simulink model "qamnrzbw"  (Simulink 7.4)
settings: Solver=ode45  StartTime=0.0  StopTime=999999  MaxStep=.05  MinStep=0.0001  RelTol=1e-6  AbsTol=1e-6
undefined symbols (not defined in the file or in its folder): eyediasi, eyesampl, sbiterr
libraries: librnew x3
CloseFcn:
  | closemodcross
settings Model: Creator=gerhard  LastModifiedBy=simulink  ExtModeAutoUpdateStatusClock=off
settings DataIOCC: SaveOutput=off  SaveTime=off  SignalLoggingName=sigsOut
settings OptimizationCC: BlockReduction=off  BooleanDataType=off
settings DebuggingCC: SaveWithParameterizedLinksMsg=none  SignalResolutionControl=TryResolveAllWithWarning  SolverPrmCheckMsg=none  MultiTaskDSMMsg=warning  MultiTaskCondExecSysMsg=none  StrictBusMsg=None
settings HardwareCC: TargetUnknown=on
settings RTWCC: IncludeERTFirstTime=on

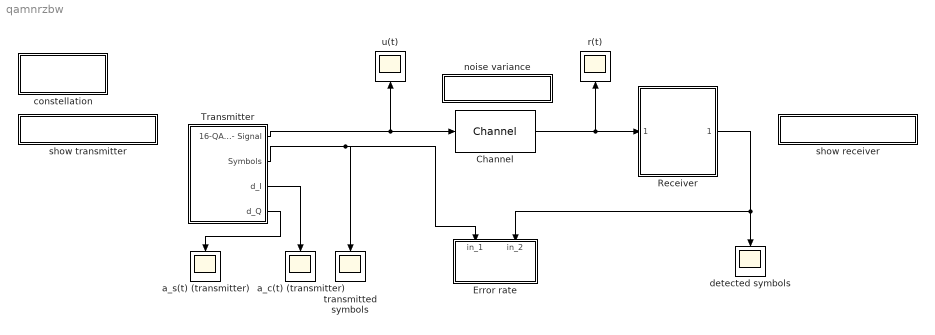
== system qamnrzbw ==
  Channel : librnew/Channel  SystemSampleTime=-1  m=0  variance=0.001  s=12345
  Error rate : Subsystem  LoadFcn=sbiterr([],[],[],'LoadBlock')  StartFcn=sbiterr([],[],[],'Start')  StopFcn=sbiterr([],[],[],'Stop')  mask(Symbol/bit error counter){@1=4, @2=10, @3=1, @4=1}
      mask prompts: @1 "Bit per symbol:"; @2 "Number of digits on display:"; @3 "Delay between 1st port and 2nd port:"; @4 "Sample time (sec):"
      mask help: Use the input data from the 1st port as the reference signal to detect the number of errors and error rate of the 2nd signal.
      mask init:
      | K=@1;num_lin=@2;TDelay=@3;Sample=@4;
      settings: CopyFcn=sbiterr([],[],[],'CopyBlock')  DeleteFcn=sbiterr([],[],[],'DeleteBlock')  NameChangeFcn=sbiterr([],[],[],'NameChange')
      mask Help: The signal from the first port must be a scalar. The second input port can be a vector with a delay to the first port signal. The comparison happens only at the sampling point.
      mask Display: disp('Error\nmeter')
  Receiver : Subsystem
  Transmitter : Subsystem
  a_c(t) (transmitter) : Scope
      settings: TimeRange=25.000000  YMin=-1.5  YMax=1.5  DataFormat=Array
  a_s(t) (transmitter) : Scope
      settings: TimeRange=25.000000  YMin=-1.5  YMax=1.5  DataFormat=Array
  constellation : Subsystem
      settings: OpenFcn=cplotqam(16)
      mask Type: constellation
      mask Display: disp('Signal Space \n Constellation')
  detected symbols : Scope
      settings: TimeRange=25.000000  YMin=-15  YMax=15  DataFormat=Array
  noise variance : Subsystem
      settings: OpenFcn=setnoise
      mask Type: noise
      mask Display: disp('Noise variance')
  r(t) : Scope
      settings: TimeRange=25.000000  YMin=-1.5  YMax=1.5  DataFormat=Array
  show receiver : Subsystem
      settings: OpenFcn=showqamr
      mask Type: open
      mask Display: disp('Receiver')
  show transmitter : Subsystem
      settings: OpenFcn=showqamt
      mask Type: open
      mask Display: disp('Transmitter')
  transmitted symbols : Scope
      settings: TimeRange=25.000000  YMin=-15  YMax=15  DataFormat=Array
  u(t) : Scope
      settings: TimeRange=25.000000  YMin=-1.5  YMax=1.5  DataFormat=Array
  wires:
  Transmitter/1(16-QAM- Signal) -> u(t)/1, Channel/1
  Channel/1 -> Receiver/1(noisy 16-QAM signal), r(t)/1
  Receiver/1(detected symbols) -> detected symbols/1, Error rate/2(in_2)
  Transmitter/4(d_Q) -> a_s(t) (transmitter)/1
  Transmitter/3(d_I) -> a_c(t) (transmitter)/1
  Transmitter/2(Symbols) -> Error rate/1(in_1), transmitted symbols/1

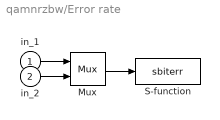
== system qamnrzbw/Error rate ==
  in_1 : Inport  OutDataType=sfix(16)  OutScaling=2^0
  in_2 : Inport  Port=2  OutDataType=sfix(16)  OutScaling=2^0
  Mux : Mux  Inputs=2
  S-function : S-Function  FunctionName=sbiterr  Parameters=num_lin, K, TDelay, Sample  EnableBusSupport=off
  wires:
  Mux/1 -> S-function/1
  in_1/1 -> Mux/1
  in_2/1 -> Mux/2

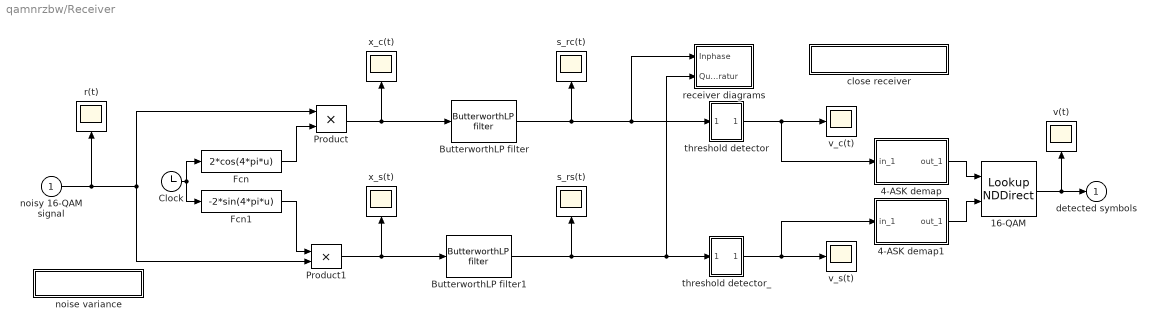
== system qamnrzbw/Receiver ==
  noisy 16-QAM signal : Inport  OutDataType=sfix(16)  OutScaling=2^0
  16-QAM : LookupNDDirect  Table=[0 1 2 3; 4 5 6 7; 8 9 10 11; 12 13 14 15]
  4-ASK demap : Subsystem  mask(MASK demapping){N=4, td=[1, .9]}
      mask prompts: N "M-ary number (digit integers in ranger [0, M-1]):"; td "Output symbol interval and offset (sec):"
      mask help:
      | Reverse the MASK mapping process
      | Convert [-1 1] analog signal to [0, M-1] symbols.
      mask init:
      | Ac=1;sft=[0:N-1]*Ac*2/(N-1)-Ac;
      mask Help: This block demaps a MASK mapped signal back to digit symbols. You can place this block after a amplitude demodulation block. The input of this block is an analog signal in the range [-1, 1]. The demodulation decides the closest integer fitting in [0,M-1] range. When the input symbol interval is a two-elements vector, the second element is offset. The default offset value is 0.
      mask Display: disp('MASK\ndemapping')
  4-ASK demap1 : Subsystem  mask(MASK demapping){N=4, td=[1, .9]}
      mask prompts: N "M-ary number (digit integers in ranger [0, M-1]):"; td "Output symbol interval and offset (sec):"
      mask help:
      | Reverse the MASK mapping process
      | Convert [-1 1] analog signal to [0, M-1] symbols.
      mask init:
      | Ac=1;sft=[0:N-1]*Ac*2/(N-1)-Ac;
      mask Help: This block demaps a MASK mapped signal back to digit symbols. You can place this block after a amplitude demodulation block. The input of this block is an analog signal in the range [-1, 1]. The demodulation decides the closest integer fitting in [0,M-1] range. When the input symbol interval is a two-elements vector, the second element is offset. The default offset value is 0.
      mask Display: disp('MASK\ndemapping')
  ButterworthLP filter : librnew/ButterworthLP filter  SystemSampleTime=-1  n=4  MaskParam1=5
  ButterworthLP filter1 : librnew/ButterworthLP filter  SystemSampleTime=-1  n=4  MaskParam1=5
  Clock : Clock
      settings: Decimation=10
  Fcn : Fcn  Expr=2*cos(4*pi*u)
  Fcn1 : Fcn  Expr=-2*sin(4*pi*u)
  Product : Product  OutDataType=sfix(16)  OutScaling=2^0  SaturateOnIntegerOverflow=on  InputSameDT=on  OutDataTypeStr=Inherit: Same as first input
  Product1 : Product  OutDataType=sfix(16)  OutScaling=2^0  SaturateOnIntegerOverflow=on  InputSameDT=on  OutDataTypeStr=Inherit: Same as first input
  close receiver : Subsystem
      settings: OpenFcn=closqamr
      mask Type: close
      mask Display: disp('close receiver')
  noise variance : Subsystem
      settings: OpenFcn=setnoise
      mask Type: noise
      mask Display: disp('Noise variance')
  r(t) : Scope
      settings: TimeRange=25.000000  YMin=-1.500000  YMax=1.500000  DataFormat=Array
  receiver diagrams : Subsystem  mask(2D-Diagrams){starttime=1, anzahl=40, offset=0.075}
      mask prompts: starttime "Plot start time:"; anzahl "Samples per time slot (2*T):"; offset "Decision offset:"
      mask help: Eye pattern, signal space trajectory and scatter plot
      mask init:
      | [x, y] = srcsicon(10);
      mask Display: plot(0,0,100,100,x,y)
  s_rc(t) : Scope
      settings: TimeRange=25.000000  YMin=-1.500000  YMax=1.500000  DataFormat=Array
  s_rs(t) : Scope
      settings: TimeRange=25.000000  YMin=-1.500000  YMax=1.500000  DataFormat=Array
  threshold detector : Subsystem
  threshold detector_ : Subsystem
  v(t) : Scope
      settings: TimeRange=25.000000  YMin=-15.000000  YMax=15.000000  DataFormat=Array
  v_c(t) : Scope
      settings: TimeRange=25.000000  YMin=-1.500000  YMax=1.500000  DataFormat=Array
  v_s(t) : Scope
      settings: TimeRange=25.000000  YMin=-1.500000  YMax=1.500000  DataFormat=Array
  x_c(t) : Scope
      settings: TimeRange=25.000000  YMin=-1.500000  YMax=1.500000  DataFormat=Array
  x_s(t) : Scope
      settings: TimeRange=25.000000  YMin=-1.500000  YMax=1.500000  DataFormat=Array
  detected symbols : Outport
  wires:
  Clock/1 -> Fcn/1, Fcn1/1
  Product/1 -> x_c(t)/1, ButterworthLP filter/1
  Product1/1 -> x_s(t)/1, ButterworthLP filter1/1
  noisy 16-QAM signal/1 -> r(t)/1, Product/1, Product1/2
  Fcn1/1 -> Product1/1
  Fcn/1 -> Product/2
  ButterworthLP filter/1 -> s_rc(t)/1, receiver diagrams/1(Inphase), threshold detector/1(in_1)
  ButterworthLP filter1/1 -> s_rs(t)/1, receiver diagrams/2(Quadratur), threshold detector_/1(in_1)
  threshold detector/1(out_1) -> v_c(t)/1, 4-ASK demap/1(in_1)
  threshold detector_/1(out_1) -> v_s(t)/1, 4-ASK demap1/1(in_1)
  4-ASK demap/1(out_1) -> 16-QAM/1
  4-ASK demap1/1(out_1) -> 16-QAM/2
  16-QAM/1 -> detected symbols/1, v(t)/1

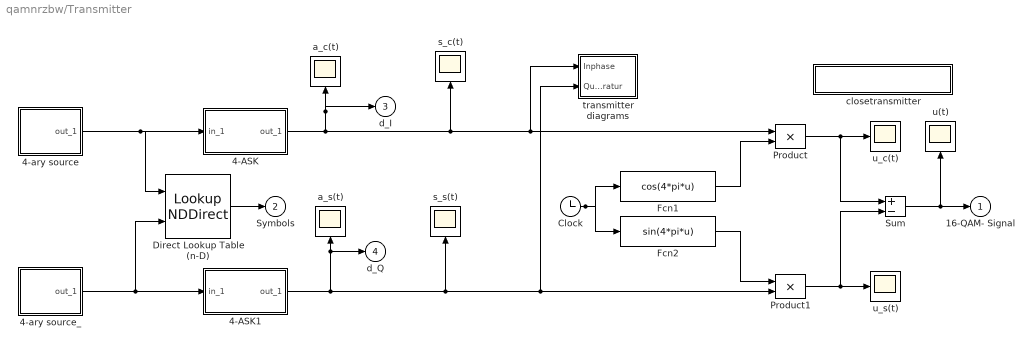
== system qamnrzbw/Transmitter ==
  4-ASK : Subsystem  mask(M-ASK mapping){N=4, td=1}
      mask prompts: N "M-ary number (input integers in range [0, M-1]):"; td "Input symbol interval and offset (sec):"
      mask help:
      | Map a digital symbol onto an analog
      | signal in the range [-1, 1] using M-ary
      | amplitude shift keying modulation mapping.
      mask init:
      | Ac=1;Kc=Ac*2/(N-1);
      mask Help: This block maps an input digit signal onto a signal in the range [-1, 1]. The coded signal can be modulated using analog\nmodulation blocks. Input digits are in the range [0, M-1], where M is the M-ary number. The input symbol interval can be a two-element vector with the second element being offset. The default value offset is 0. Use the MODMAP function to see the constellation.
      mask Display: disp('MASK\nmapping')
  4-ASK1 : Subsystem  mask(M-ASK mapping){N=4, td=1}
      mask prompts: N "M-ary number (input integers in range [0, M-1]):"; td "Input symbol interval and offset (sec):"
      mask help:
      | Map a digital symbol onto an analog
      | signal in the range [-1, 1] using M-ary
      | amplitude shift keying modulation mapping.
      mask init:
      | Ac=1;Kc=Ac*2/(N-1);
      mask Help: This block maps an input digit signal onto a signal in the range [-1, 1]. The coded signal can be modulated using analog\nmodulation blocks. Input digits are in the range [0, M-1], where M is the M-ary number. The input symbol interval can be a two-element vector with the second element being offset. The default value offset is 0. Use the MODMAP function to see the constellation.
      mask Display: disp('MASK\nmapping')
  4-ary source : Subsystem  mask(Read from workspace){@1=randint(2000,1,4), @2=1, @3=1, @4=1}
      mask prompts: @1 "Variable (column_number=block_output_length):"; @2 "Data output sample time (sec):"; @3 "Repeat flag (1: repeat read, 0: output zeros after eof)."; @4 "Initial output:"
      mask help:
      | Read from a workspace variable at
      | sampling time point.
      mask init:
      | var=@1;td=@2;ts=td(1);if (length(td)>=2),off=td(2);else off=0;end;cyc=@3;ini=@4;[x,y]=srcsicon(7);
      mask Help: This block reads from a workspace variable at a given sample time. The column number is the block output vector length. When the simulation reaches the end of the variable (eof), the block will cyclically output from the first row of the variable or output zeros based on the repeat flag entree.
      mask Display: plot(0,0,100,100,x,y);disp('Rd wksp')
  4-ary source_ : Subsystem  mask(Read from workspace){@1=randint(2000,1,4), @2=1, @3=1, @4=1}
      mask prompts: @1 "Variable (column_number=block_output_length):"; @2 "Data output sample time (sec):"; @3 "Repeat flag (1: repeat read, 0: output zeros after eof)."; @4 "Initial output:"
      mask help:
      | Read from a workspace variable at
      | sampling time point.
      mask init:
      | var=@1;td=@2;ts=td(1);if (length(td)>=2),off=td(2);else off=0;end;cyc=@3;ini=@4;[x,y]=srcsicon(7);
      mask Help: This block reads from a workspace variable at a given sample time. The column number is the block output vector length. When the simulation reaches the end of the variable (eof), the block will cyclically output from the first row of the variable or output zeros based on the repeat flag entree.
      mask Display: plot(0,0,100,100,x,y);disp('Rd wksp')
  Clock : Clock
      settings: Decimation=10
  Direct Lookup Table (n-D) : LookupNDDirect  Table=[0 1 2 3; 4 5 6 7; 8 9 10 11; 12 13 14 15]
  Fcn1 : Fcn  Expr=cos(4*pi*u)
  Fcn2 : Fcn  Expr=sin(4*pi*u)
  Product : Product  OutDataType=sfix(16)  OutScaling=2^0  SaturateOnIntegerOverflow=on  InputSameDT=on  OutDataTypeStr=Inherit: Same as first input
  Product1 : Product  OutDataType=sfix(16)  OutScaling=2^0  SaturateOnIntegerOverflow=on  InputSameDT=on  OutDataTypeStr=Inherit: Same as first input
  Sum : Sum  Inputs=+-  OutDataType=sfix(16)  OutScaling=2^0  SaturateOnIntegerOverflow=on  InputSameDT=on  OutDataTypeStr=Inherit: Same as first input
  a_c(t) : Scope
      settings: TimeRange=25.000000  YMin=-1.500000  YMax=1.500000  DataFormat=Array
  a_s(t) : Scope
      settings: TimeRange=25.000000  YMin=-1.500000  YMax=1.500000  DataFormat=Array
  closetransmitter : Subsystem
      settings: OpenFcn=closetra
      mask Type: close
      mask Display: disp('Close transmitter')
  s_c(t) : Scope
      settings: TimeRange=25.000000  YMin=-1.500000  YMax=1.500000  DataFormat=Array
  s_s(t) : Scope
      settings: TimeRange=25.000000  YMin=-1.500000  YMax=1.500000  DataFormat=Array
  transmitter diagrams : Subsystem  mask(2D-Diagrams){starttime=0, anzahl=40, offset=0}
      mask prompts: starttime "Plot start time:"; anzahl "Samples per time slot (2*T):"; offset "Decision offset:"
      mask help: Eye pattern, signal space trajectory and scatter plot
      mask init:
      | [x, y] = srcsicon(10);
      mask Display: plot(0,0,100,100,x,y)
  u(t) : Scope
      settings: TimeRange=25.000000  YMin=-1.500000  YMax=1.500000  DataFormat=Array
  u_c(t) : Scope
      settings: TimeRange=25.000000  YMin=-1.500000  YMax=1.500000  DataFormat=Array
  u_s(t) : Scope
      settings: TimeRange=25.000000  YMin=-1.500000  YMax=1.500000  DataFormat=Array
  16-QAM- Signal : Outport
  Symbols : Outport  Port=2
  d_I : Outport  Port=3
  d_Q : Outport  Port=4
  wires:
  Product1/1 -> u_s(t)/1, Sum/2
  Product/1 -> u_c(t)/1, Sum/1
  Clock/1 -> Fcn2/1, Fcn1/1
  Fcn1/1 -> Product/2
  Fcn2/1 -> Product1/1
  Sum/1 -> u(t)/1, 16-QAM- Signal/1
  4-ary source/1(out_1) -> 4-ASK/1(in_1), Direct Lookup Table (n-D)/1
  Direct Lookup Table (n-D)/1 -> Symbols/1
  4-ASK/1(out_1) -> a_c(t)/1, d_I/1, Product/1, transmitter diagrams/1(Inphase), s_c(t)/1
  4-ASK1/1(out_1) -> a_s(t)/1, d_Q/1, s_s(t)/1, Product1/2, transmitter diagrams/2(Quadratur)
  4-ary source_/1(out_1) -> 4-ASK1/1(in_1), Direct Lookup Table (n-D)/2

== system qamnrzbw/constellation ==

== system qamnrzbw/noise variance ==

== system qamnrzbw/show receiver ==

== system qamnrzbw/show transmitter ==

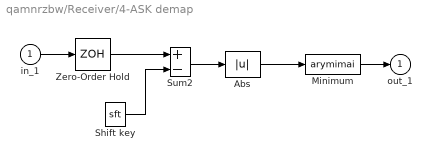
== system qamnrzbw/Receiver/4-ASK demap ==
  in_1 : Inport  OutDataType=sfix(16)  OutScaling=2^0
  Abs : Abs  SaturateOnIntegerOverflow=on
  Minimum : S-Function  FunctionName=arymimai  Parameters='min'  EnableBusSupport=off
  Shift key : Constant  Value=sft  OutDataType=sfix(16)  OutScaling=2^0
  Sum2 : Sum  Inputs=+-  OutDataType=sfix(16)  OutScaling=2^0  SaturateOnIntegerOverflow=on  InputSameDT=on  OutDataTypeStr=Inherit: Same as first input
  Zero-Order Hold : ZeroOrderHold  SampleTime=td
  out_1 : Outport
  wires:
  Sum2/1 -> Abs/1
  Shift key/1 -> Sum2/2
  Minimum/1 -> out_1/1
  Zero-Order Hold/1 -> Sum2/1
  Abs/1 -> Minimum/1
  in_1/1 -> Zero-Order Hold/1

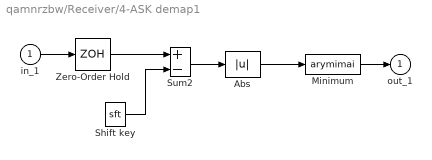
== system qamnrzbw/Receiver/4-ASK demap1 ==
  in_1 : Inport  OutDataType=sfix(16)  OutScaling=2^0
  Abs : Abs  SaturateOnIntegerOverflow=on
  Minimum : S-Function  FunctionName=arymimai  Parameters='min'  EnableBusSupport=off
  Shift key : Constant  Value=sft  OutDataType=sfix(16)  OutScaling=2^0
  Sum2 : Sum  Inputs=+-  OutDataType=sfix(16)  OutScaling=2^0  SaturateOnIntegerOverflow=on  InputSameDT=on  OutDataTypeStr=Inherit: Same as first input
  Zero-Order Hold : ZeroOrderHold  SampleTime=td
  out_1 : Outport
  wires:
  Sum2/1 -> Abs/1
  Shift key/1 -> Sum2/2
  Minimum/1 -> out_1/1
  Zero-Order Hold/1 -> Sum2/1
  Abs/1 -> Minimum/1
  in_1/1 -> Zero-Order Hold/1

== system qamnrzbw/Receiver/close receiver ==

== system qamnrzbw/Receiver/noise variance ==

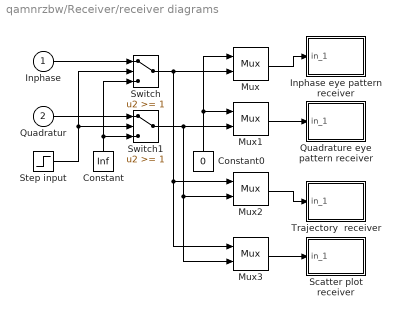
== system qamnrzbw/Receiver/receiver diagrams ==
  Inphase : Inport  OutDataType=sfix(16)  OutScaling=2^0
  Quadratur : Inport  Port=2  OutDataType=sfix(16)  OutScaling=2^0
  Constant : Constant  Value=Inf  OutDataType=sfix(16)  OutScaling=2^0
  Constant0 : Constant  Value=0  OutDataType=sfix(16)  OutScaling=2^0
  Inphase eye pattern receiver : Subsystem  LoadFcn=eyesampl([],[],[],'LoadBlock')  StartFcn=eyesampl([],[],[],'Start')  StopFcn=eyesampl([],[],[],'Stop')  mask(Eye-diagram/scatter plot){@1=[2 0 1+offset], @2=[-1.5 1.5], @3=0, @4='w-/r-', @5=0, @6=2/anzahl}
      mask prompts: @1 "[Symbol interval, plot offset, decision point offset]:"; @2 "Lower and upper bound of in-coming signal (1x2 vector):"; @3 "Number of saved traces:"; @4 "Line-type for eye-pattern diagram (0 for no plot):"; @5 "Line-type for scatter plot (0 for no plot):"; @6 "Plot update sample time:"
      mask help: Produce eye-pattern diagram and/or scatter plot.
      mask init:
      | time_range=@1;boundary=@2;kept_length=@3;eye_line=@4;scatter_line=@5;two_d_line=@6;[x,y]=srcsicon(10);
      settings: CopyFcn=eyesampl([],[],[],'CopyBlock')  DeleteFcn=eyesampl([],[],[],'DeleteBlock')  NameChangeFcn=eyesampl([],[],[],'NameChange')
      mask Help: This plot opens one, or two plots by assigning the line type parameters. The scatter plot point is selected by the decision point in the first parameter entry. A decision line is drawn in the eye-pattern diagram. The plot is updated at the plot update sample time point.
      mask Display: plot(0,0,100,100,x,y);
  Mux{,1..3} (4 alike) : Mux  Inputs=2
  Quadrature eye pattern receiver : Subsystem  LoadFcn=eyesampl([],[],[],'LoadBlock')  StartFcn=eyesampl([],[],[],'Start')  StopFcn=eyesampl([],[],[],'Stop')  mask(Eye-diagram/scatter plot){@1=[2 0 1+offset], @2=[-1.5 1.5], @3=0, @4='w-/r-', @5=0, @6=2/anzahl}
      mask prompts: @1 "[Symbol interval, plot offset, decision point offset]:"; @2 "Lower and upper bound of in-coming signal (1x2 vector):"; @3 "Number of saved traces:"; @4 "Line-type for eye-pattern diagram (0 for no plot):"; @5 "Line-type for scatter plot (0 for no plot):"; @6 "Plot update sample time:"
      mask help: Produce eye-pattern diagram and/or scatter plot.
      mask init:
      | time_range=@1;boundary=@2;kept_length=@3;eye_line=@4;scatter_line=@5;two_d_line=@6;[x,y]=srcsicon(10);
      settings: CopyFcn=eyesampl([],[],[],'CopyBlock')  DeleteFcn=eyesampl([],[],[],'DeleteBlock')  NameChangeFcn=eyesampl([],[],[],'NameChange')
      mask Help: This plot opens one, or two plots by assigning the line type parameters. The scatter plot point is selected by the decision point in the first parameter entry. A decision line is drawn in the eye-pattern diagram. The plot is updated at the plot update sample time point.
      mask Display: plot(0,0,100,100,x,y);
  Scatter plot receiver : Subsystem  LoadFcn=eyesampl([],[],[],'LoadBlock')  StartFcn=eyesampl([],[],[],'Start')  StopFcn=eyesampl([],[],[],'Stop')  mask(Eye-diagram/scatter plot){@1=[1 .5 .999], @2=[-1.5 1.5], @3=0, @4=0, @5='b.', @6=[.5 offset]}
      mask prompts: @1 "[Symbol interval, plot offset, decision point offset]:"; @2 "Lower and upper bound of in-coming signal (1x2 vector):"; @3 "Number of saved traces:"; @4 "Line-type for eye-pattern diagram (0 for no plot):"; @5 "Line-type for scatter plot (0 for no plot):"; @6 "Plot update sample time:"
      mask help: Produce eye-pattern diagram and/or scatter plot.
      mask init:
      | time_range=@1;boundary=@2;kept_length=@3;eye_line=@4;scatter_line=@5;two_d_line=@6;[x,y]=srcsicon(10);
      settings: CopyFcn=eyesampl([],[],[],'CopyBlock')  DeleteFcn=eyesampl([],[],[],'DeleteBlock')  NameChangeFcn=eyesampl([],[],[],'NameChange')
      mask Help: This plot opens one, or two plots by assigning the line type parameters. The scatter plot point is selected by the decision point in the first parameter entry. A decision line is drawn in the eye-pattern diagram. The plot is updated at the plot update sample time point.
      mask Display: plot(0,0,100,100,x,y);
  Step input : Step  Time=starttime  SampleTime=1
  Switch : Switch  Threshold=1  SaturateOnIntegerOverflow=on  InputSameDT=on
  Switch1 : Switch  Threshold=1  SaturateOnIntegerOverflow=on  InputSameDT=on
  Trajectory  receiver : Subsystem  LoadFcn=eyediasi([],[],[],'LoadBlock')  StartFcn=eyediasi([],[],[],'Start')  StopFcn=eyediasi([],[],[],'Stop')  mask(Eye-diagram/scatter plot){@1=[2 0 1], @2=[-1.5 1.5], @3=0, @4=0, @5=0, @6='g-'}
      mask prompts: @1 "Eye-pattern plot time frame:"; @2 "Lower and upper bound of in-coming signal (1x2 vector):"; @3 "Number of saved traces:"; @4 "Line-type for eye-pattern diagram (0 for no plot):"; @5 "Line-type for scatter plot (0 for no plot):"; @6 "Line-type for x-y plot (0 for no plot):"
      mask help:
      | Produce eye-pattern diagram/scatter
      | plot/x-y plot with the rising edge of the second input as the decision line.
      mask init:
      | time_range=@1;boundary=@2;kept_length=@3;eye_line=@4;scatter_line=@5;two_d_line=@6;[x,y]=srcsicon(10);[v,w]=trigicon(0,25,get_param(gcb,'orientation'),2);
      settings: CopyFcn=eyediasi([],[],[],'CopyBlock')  DeleteFcn=eyediasi([],[],[],'DeleteBlock')  NameChangeFcn=eyediasi([],[],[],'NameChange')
      mask Help: This plot opens one, two, or three plots by assigning the line type parameters. The scatter plot point is selected by the rising edge of a trigger signal. A decision line is drawn at the rising edge of the trigger signal.
      mask Display: plot(0,0,100,100,x,y,v,w);
  wires:
  Switch/1 -> Mux/2, Mux3/1, Mux2/1
  Switch1/1 -> Mux1/2, Mux3/2, Mux2/2
  Constant0/1 -> Mux1/1, Mux/1
  Quadratur/1 -> Switch1/1
  Inphase/1 -> Switch/1
  Step input/1 -> Switch/2, Switch1/2
  Constant/1 -> Switch/3, Switch1/3
  Mux1/1 -> Quadrature eye pattern receiver/1(in_1)
  Mux/1 -> Inphase eye pattern receiver/1(in_1)
  Mux3/1 -> Scatter plot receiver/1(in_1)
  Mux2/1 -> Trajectory  receiver/1(in_1)

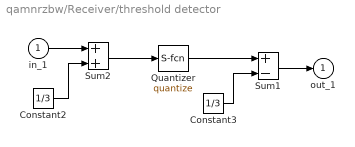
== system qamnrzbw/Receiver/threshold detector ==
  in_1 : Inport  OutDataType=sfix(16)  OutScaling=2^0
  Constant2 : Constant  Value=1/3  OutDataType=sfix(16)  OutScaling=2^0
  Constant3 : Constant  Value=1/3  OutDataType=sfix(16)  OutScaling=2^0
  Quantizer : S-Function  FunctionName=quantize  Parameters=q  EnableBusSupport=off  mask(Quantizer){@1=2/3}
      mask prompts: @1 "Quantization interval:"
      mask help: Discretizes input at given interval.
      mask init:
      | q = @1;
      mask Help: Quantizes input in given intervals.
      mask Display: plot([-4,4],[0,0],[0,0],[-4,4],[-3,-2,-2,-1,-1,0,0,1,1,2,2,3,3,4]-0.5,[-3,-3,-2,-2,-1,-1,0,0,1,1,2,2,3,3])
  Sum1 : Sum  Inputs=+-  OutDataType=sfix(16)  OutScaling=2^0  SaturateOnIntegerOverflow=on  InputSameDT=on  OutDataTypeStr=Inherit: Same as first input
  Sum2 : Sum  OutDataType=sfix(16)  OutScaling=2^0  SaturateOnIntegerOverflow=on  InputSameDT=on  OutDataTypeStr=Inherit: Same as first input
  out_1 : Outport
  wires:
  in_1/1 -> Sum2/1
  Sum2/1 -> Quantizer/1
  Constant2/1 -> Sum2/2
  Quantizer/1 -> Sum1/1
  Constant3/1 -> Sum1/2
  Sum1/1 -> out_1/1

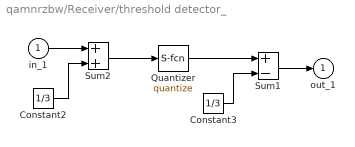
== system qamnrzbw/Receiver/threshold detector_ ==
  in_1 : Inport  OutDataType=sfix(16)  OutScaling=2^0
  Constant2 : Constant  Value=1/3  OutDataType=sfix(16)  OutScaling=2^0
  Constant3 : Constant  Value=1/3  OutDataType=sfix(16)  OutScaling=2^0
  Quantizer : S-Function  FunctionName=quantize  Parameters=q  EnableBusSupport=off  mask(Quantizer){@1=2/3}
      mask prompts: @1 "Quantization interval:"
      mask help: Discretizes input at given interval.
      mask init:
      | q = @1;
      mask Help: Quantizes input in given intervals.
      mask Display: plot([-4,4],[0,0],[0,0],[-4,4],[-3,-2,-2,-1,-1,0,0,1,1,2,2,3,3,4]-0.5,[-3,-3,-2,-2,-1,-1,0,0,1,1,2,2,3,3])
  Sum1 : Sum  Inputs=+-  OutDataType=sfix(16)  OutScaling=2^0  SaturateOnIntegerOverflow=on  InputSameDT=on  OutDataTypeStr=Inherit: Same as first input
  Sum2 : Sum  OutDataType=sfix(16)  OutScaling=2^0  SaturateOnIntegerOverflow=on  InputSameDT=on  OutDataTypeStr=Inherit: Same as first input
  out_1 : Outport
  wires:
  Sum1/1 -> out_1/1
  Constant3/1 -> Sum1/2
  Quantizer/1 -> Sum1/1
  Constant2/1 -> Sum2/2
  Sum2/1 -> Quantizer/1
  in_1/1 -> Sum2/1

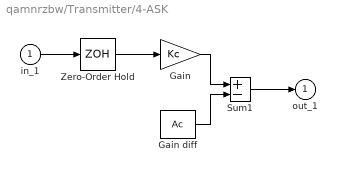
== system qamnrzbw/Transmitter/4-ASK ==
  in_1 : Inport  OutDataType=sfix(16)  OutScaling=2^0
  Gain : Gain  Gain=Kc  ParameterDataType=sfix(16)  ParameterScaling=2^0  OutDataType=sfix(16)  OutScaling=2^0  SaturateOnIntegerOverflow=on  OutDataTypeStr=Inherit: Same as input  ParamDataTypeStr=Inherit: Same as input
  Gain diff : Constant  Value=Ac  OutDataType=sfix(16)  OutScaling=2^0
  Sum1 : Sum  Inputs=+-  OutDataType=sfix(16)  OutScaling=2^0  SaturateOnIntegerOverflow=on  InputSameDT=on  OutDataTypeStr=Inherit: Same as first input
  Zero-Order Hold : ZeroOrderHold  SampleTime=td
  out_1 : Outport
  wires:
  Zero-Order Hold/1 -> Gain/1
  in_1/1 -> Zero-Order Hold/1
  Sum1/1 -> out_1/1
  Gain diff/1 -> Sum1/2
  Gain/1 -> Sum1/1

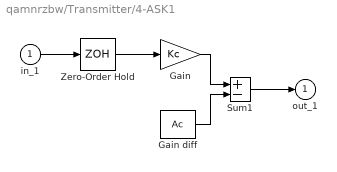
== system qamnrzbw/Transmitter/4-ASK1 ==
  in_1 : Inport  OutDataType=sfix(16)  OutScaling=2^0
  Gain : Gain  Gain=Kc  ParameterDataType=sfix(16)  ParameterScaling=2^0  OutDataType=sfix(16)  OutScaling=2^0  SaturateOnIntegerOverflow=on  OutDataTypeStr=Inherit: Same as input  ParamDataTypeStr=Inherit: Same as input
  Gain diff : Constant  Value=Ac  OutDataType=sfix(16)  OutScaling=2^0
  Sum1 : Sum  Inputs=+-  OutDataType=sfix(16)  OutScaling=2^0  SaturateOnIntegerOverflow=on  InputSameDT=on  OutDataTypeStr=Inherit: Same as first input
  Zero-Order Hold : ZeroOrderHold  SampleTime=td
  out_1 : Outport
  wires:
  Gain/1 -> Sum1/1
  Gain diff/1 -> Sum1/2
  Sum1/1 -> out_1/1
  in_1/1 -> Zero-Order Hold/1
  Zero-Order Hold/1 -> Gain/1

== system qamnrzbw/Transmitter/4-ary source ==
  Message source : S-Function  FunctionName=trigwksp  Parameters=var,thd,cyclFlag,ini  EnableBusSupport=off  mask(Read from workspace){@1=var, @2=.1, @3=cyc, @4=ini}
      mask prompts: @1 "Read the variable:"; @2 "Threshold for the input pulse:"; @3 "Cyclic read variable (1) or amend zeros (0)."; @4 "Output before first trigger:"
      mask help: The raising edge of input pulse trigger the block output the next row from the workspace variable.
      mask init:
      | var=@1;thd=@2;cyclFlag=@3;ini=@4;
      mask Help: This block reads the data from a workspace variable. The output is refreshed at the raising edge of the input pulse.
      mask Display: disp('Triggered\nread')
  Pulses deivide same sample time1 : Subsystem  mask(Pulse generator){@1=ts, @2=1, @3=off}
      mask prompts: @1 "Sample time (scalar, sec):"; @2 "Divider (integer vector):"; @3 "Offset (have same dimension as Divider:"
      mask help: Vector pulses with sample rate of each pulse as Sample_time ./Divider.
      mask init:
      | samp_time=@1;out_divid=@2;offset=@3;
      mask Help: This block generator a vector pulses. The output length is the same as the vector defined in "Divider". The ith element of the output has the sample time Sample_time/Divider(i). All elements in "Divider" must be integers.
      mask Display: disp('Vector\nPulse')
  out_1 : Outport
  wires:
  Pulses deivide same sample time1/1(Outport) -> Message source/1
  Message source/1 -> out_1/1

== system qamnrzbw/Transmitter/4-ary source_ ==
  Message source : S-Function  FunctionName=trigwksp  Parameters=var,thd,cyclFlag,ini  EnableBusSupport=off  mask(Read from workspace){@1=var, @2=.1, @3=cyc, @4=ini}
      mask prompts: @1 "Read the variable:"; @2 "Threshold for the input pulse:"; @3 "Cyclic read variable (1) or amend zeros (0)."; @4 "Output before first trigger:"
      mask help: The raising edge of input pulse trigger the block output the next row from the workspace variable.
      mask init:
      | var=@1;thd=@2;cyclFlag=@3;ini=@4;
      mask Help: This block reads the data from a workspace variable. The output is refreshed at the raising edge of the input pulse.
      mask Display: disp('Triggered\nread')
  Pulses deivide same sample time1 : Subsystem  mask(Pulse generator){@1=ts, @2=1, @3=off}
      mask prompts: @1 "Sample time (scalar, sec):"; @2 "Divider (integer vector):"; @3 "Offset (have same dimension as Divider:"
      mask help: Vector pulses with sample rate of each pulse as Sample_time ./Divider.
      mask init:
      | samp_time=@1;out_divid=@2;offset=@3;
      mask Help: This block generator a vector pulses. The output length is the same as the vector defined in "Divider". The ith element of the output has the sample time Sample_time/Divider(i). All elements in "Divider" must be integers.
      mask Display: disp('Vector\nPulse')
  out_1 : Outport
  wires:
  Pulses deivide same sample time1/1(Outport) -> Message source/1
  Message source/1 -> out_1/1

== system qamnrzbw/Transmitter/closetransmitter ==

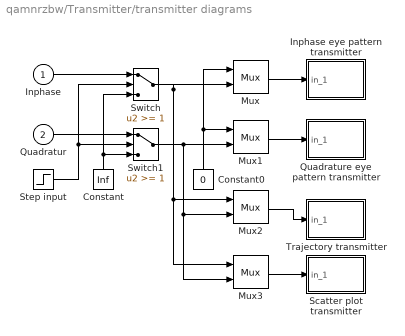
== system qamnrzbw/Transmitter/transmitter diagrams ==
  Inphase : Inport  OutDataType=sfix(16)  OutScaling=2^0
  Quadratur : Inport  Port=2  OutDataType=sfix(16)  OutScaling=2^0
  Constant : Constant  Value=Inf  OutDataType=sfix(16)  OutScaling=2^0
  Constant0 : Constant  Value=0  OutDataType=sfix(16)  OutScaling=2^0
  Inphase eye pattern transmitter : Subsystem  LoadFcn=eyesampl([],[],[],'LoadBlock')  StartFcn=eyesampl([],[],[],'Start')  StopFcn=eyesampl([],[],[],'Stop')  mask(Eye-diagram/scatter plot){@1=[2 0 1+offset], @2=[-1.5 1.5], @3=0, @4='w-/r-', @5=0, @6=2/anzahl}
      mask prompts: @1 "[Symbol interval, plot offset, decision point offset]:"; @2 "Lower and upper bound of in-coming signal (1x2 vector):"; @3 "Number of saved traces:"; @4 "Line-type for eye-pattern diagram (0 for no plot):"; @5 "Line-type for scatter plot (0 for no plot):"; @6 "Plot update sample time:"
      mask help: Produce eye-pattern diagram and/or scatter plot.
      mask init:
      | time_range=@1;boundary=@2;kept_length=@3;eye_line=@4;scatter_line=@5;two_d_line=@6;[x,y]=srcsicon(10);
      settings: CopyFcn=eyesampl([],[],[],'CopyBlock')  DeleteFcn=eyesampl([],[],[],'DeleteBlock')  NameChangeFcn=eyesampl([],[],[],'NameChange')
      mask Help: This plot opens one, or two plots by assigning the line type parameters. The scatter plot point is selected by the decision point in the first parameter entry. A decision line is drawn in the eye-pattern diagram. The plot is updated at the plot update sample time point.
      mask Display: plot(0,0,100,100,x,y);
  Mux{,1..3} (4 alike) : Mux  Inputs=2
  Quadrature eye pattern transmitter : Subsystem  LoadFcn=eyesampl([],[],[],'LoadBlock')  StartFcn=eyesampl([],[],[],'Start')  StopFcn=eyesampl([],[],[],'Stop')  mask(Eye-diagram/scatter plot){@1=[2 0 1+offset], @2=[-1.5 1.5], @3=0, @4='w-/r-', @5=0, @6=2/anzahl}
      mask prompts: @1 "[Symbol interval, plot offset, decision point offset]:"; @2 "Lower and upper bound of in-coming signal (1x2 vector):"; @3 "Number of saved traces:"; @4 "Line-type for eye-pattern diagram (0 for no plot):"; @5 "Line-type for scatter plot (0 for no plot):"; @6 "Plot update sample time:"
      mask help: Produce eye-pattern diagram and/or scatter plot.
      mask init:
      | time_range=@1;boundary=@2;kept_length=@3;eye_line=@4;scatter_line=@5;two_d_line=@6;[x,y]=srcsicon(10);
      settings: CopyFcn=eyesampl([],[],[],'CopyBlock')  DeleteFcn=eyesampl([],[],[],'DeleteBlock')  NameChangeFcn=eyesampl([],[],[],'NameChange')
      mask Help: This plot opens one, or two plots by assigning the line type parameters. The scatter plot point is selected by the decision point in the first parameter entry. A decision line is drawn in the eye-pattern diagram. The plot is updated at the plot update sample time point.
      mask Display: plot(0,0,100,100,x,y);
  Scatter plot transmitter : Subsystem  LoadFcn=eyesampl([],[],[],'LoadBlock')  StartFcn=eyesampl([],[],[],'Start')  StopFcn=eyesampl([],[],[],'Stop')  mask(Eye-diagram/scatter plot){@1=[1 .5 .999], @2=[-1.5 1.5], @3=0, @4=0, @5='b.', @6=[.5 offset]}
      mask prompts: @1 "[Symbol interval, plot offset, decision point offset]:"; @2 "Lower and upper bound of in-coming signal (1x2 vector):"; @3 "Number of saved traces:"; @4 "Line-type for eye-pattern diagram (0 for no plot):"; @5 "Line-type for scatter plot (0 for no plot):"; @6 "Plot update sample time:"
      mask help: Produce eye-pattern diagram and/or scatter plot.
      mask init:
      | time_range=@1;boundary=@2;kept_length=@3;eye_line=@4;scatter_line=@5;two_d_line=@6;[x,y]=srcsicon(10);
      settings: CopyFcn=eyesampl([],[],[],'CopyBlock')  DeleteFcn=eyesampl([],[],[],'DeleteBlock')  NameChangeFcn=eyesampl([],[],[],'NameChange')
      mask Help: This plot opens one, or two plots by assigning the line type parameters. The scatter plot point is selected by the decision point in the first parameter entry. A decision line is drawn in the eye-pattern diagram. The plot is updated at the plot update sample time point.
      mask Display: plot(0,0,100,100,x,y);
  Step input : Step  Time=starttime  SampleTime=1
  Switch : Switch  Threshold=1  SaturateOnIntegerOverflow=on  InputSameDT=on
  Switch1 : Switch  Threshold=1  SaturateOnIntegerOverflow=on  InputSameDT=on
  Trajectory transmitter : Subsystem  LoadFcn=eyediasi([],[],[],'LoadBlock')  StartFcn=eyediasi([],[],[],'Start')  StopFcn=eyediasi([],[],[],'Stop')  mask(Eye-diagram/scatter plot){@1=[2 0 1], @2=[-1.5 1.5], @3=0, @4=0, @5=0, @6='g-'}
      mask prompts: @1 "Eye-pattern plot time frame:"; @2 "Lower and upper bound of in-coming signal (1x2 vector):"; @3 "Number of saved traces:"; @4 "Line-type for eye-pattern diagram (0 for no plot):"; @5 "Line-type for scatter plot (0 for no plot):"; @6 "Line-type for x-y plot (0 for no plot):"
      mask help:
      | Produce eye-pattern diagram/scatter
      | plot/x-y plot with the rising edge of the second input as the decision line.
      mask init:
      | time_range=@1;boundary=@2;kept_length=@3;eye_line=@4;scatter_line=@5;two_d_line=@6;[x,y]=srcsicon(10);[v,w]=trigicon(0,25,get_param(gcb,'orientation'),2);
      settings: CopyFcn=eyediasi([],[],[],'CopyBlock')  DeleteFcn=eyediasi([],[],[],'DeleteBlock')  NameChangeFcn=eyediasi([],[],[],'NameChange')
      mask Help: This plot opens one, two, or three plots by assigning the line type parameters. The scatter plot point is selected by the rising edge of a trigger signal. A decision line is drawn at the rising edge of the trigger signal.
      mask Display: plot(0,0,100,100,x,y,v,w);
  wires:
  Mux2/1 -> Trajectory transmitter/1(in_1)
  Mux3/1 -> Scatter plot transmitter/1(in_1)
  Mux/1 -> Inphase eye pattern transmitter/1(in_1)
  Mux1/1 -> Quadrature eye pattern transmitter/1(in_1)
  Constant/1 -> Switch/3, Switch1/3
  Step input/1 -> Switch/2, Switch1/2
  Inphase/1 -> Switch/1
  Quadratur/1 -> Switch1/1
  Switch/1 -> Mux3/1, Mux2/1, Mux/2
  Switch1/1 -> Mux3/2, Mux2/2, Mux1/2
  Constant0/1 -> Mux1/1, Mux/1

== system qamnrzbw/Receiver/receiver diagrams/Inphase eye pattern receiver ==
  in_1 : Inport  OutDataType=sfix(16)  OutScaling=2^0
  Plot1 : S-Function  FunctionName=eyesampl  Parameters=time_range, boundary, kept_length, eye_line, scatter_line, two_d_line  EnableBusSupport=off
  wires:
  in_1/1 -> Plot1/1

== system qamnrzbw/Receiver/receiver diagrams/Quadrature eye pattern receiver ==
  in_1 : Inport  OutDataType=sfix(16)  OutScaling=2^0
  Plot1 : S-Function  FunctionName=eyesampl  Parameters=time_range, boundary, kept_length, eye_line, scatter_line, two_d_line  EnableBusSupport=off
  wires:
  in_1/1 -> Plot1/1

== system qamnrzbw/Receiver/receiver diagrams/Scatter plot receiver ==
  in_1 : Inport  OutDataType=sfix(16)  OutScaling=2^0
  Plot1 : S-Function  FunctionName=eyesampl  Parameters=time_range, boundary, kept_length, eye_line, scatter_line, two_d_line  EnableBusSupport=off
  wires:
  in_1/1 -> Plot1/1

== system qamnrzbw/Receiver/receiver diagrams/Trajectory  receiver ==
  in_1 : Inport  OutDataType=sfix(16)  OutScaling=2^0
  Constant : Constant  Value=0  OutDataType=sfix(16)  OutScaling=2^0
  Mux : Mux  Inputs=2
  Plot1 : S-Function  FunctionName=eyediasi  Parameters=time_range, boundary, kept_length, eye_line, scatter_line, two_d_line  EnableBusSupport=off
  wires:
  in_1/1 -> Mux/1
  Constant/1 -> Mux/2
  Mux/1 -> Plot1/1

== system qamnrzbw/Transmitter/4-ary source/Pulses deivide same sample time1 ==
  S-function1 : S-Function  FunctionName=homopuls  Parameters=samp_time, out_divid, offset  EnableBusSupport=off
  Outport : Outport
  wires:
  S-function1/1 -> Outport/1

== system qamnrzbw/Transmitter/4-ary source_/Pulses deivide same sample time1 ==
  S-function1 : S-Function  FunctionName=homopuls  Parameters=samp_time, out_divid, offset  EnableBusSupport=off
  Outport : Outport
  wires:
  S-function1/1 -> Outport/1

== system qamnrzbw/Transmitter/transmitter diagrams/Inphase eye pattern transmitter ==
  in_1 : Inport  OutDataType=sfix(16)  OutScaling=2^0
  Plot1 : S-Function  FunctionName=eyesampl  Parameters=time_range, boundary, kept_length, eye_line, scatter_line, two_d_line  EnableBusSupport=off
  wires:
  in_1/1 -> Plot1/1

== system qamnrzbw/Transmitter/transmitter diagrams/Quadrature eye pattern transmitter ==
  in_1 : Inport  OutDataType=sfix(16)  OutScaling=2^0
  Plot1 : S-Function  FunctionName=eyesampl  Parameters=time_range, boundary, kept_length, eye_line, scatter_line, two_d_line  EnableBusSupport=off
  wires:
  in_1/1 -> Plot1/1

== system qamnrzbw/Transmitter/transmitter diagrams/Scatter plot transmitter ==
  in_1 : Inport  OutDataType=sfix(16)  OutScaling=2^0
  Plot1 : S-Function  FunctionName=eyesampl  Parameters=time_range, boundary, kept_length, eye_line, scatter_line, two_d_line  EnableBusSupport=off
  wires:
  in_1/1 -> Plot1/1

== system qamnrzbw/Transmitter/transmitter diagrams/Trajectory transmitter ==
  in_1 : Inport  OutDataType=sfix(16)  OutScaling=2^0
  Constant : Constant  Value=0  OutDataType=sfix(16)  OutScaling=2^0
  Mux : Mux  Inputs=2
  Plot1 : S-Function  FunctionName=eyediasi  Parameters=time_range, boundary, kept_length, eye_line, scatter_line, two_d_line  EnableBusSupport=off
  wires:
  Mux/1 -> Plot1/1
  Constant/1 -> Mux/2
  in_1/1 -> Mux/1
